simulink model "viatoc_run_sim"  (R2017b)
settings: Solver=FixedStepAuto  StartTime=0.0  StopTime=60  FixedStep=Ts  RelTol=1e-3
values from neighbouring files (symbols this model uses):
  Ts = 0.2    [U.mat]    (also in X.mat; hanging_chain_benchmark.m; num_iters.mat)
  u_0 = [-2 2 2]    [U.mat]    (also in X.mat; hanging_chain_benchmark.m = [-1; 1; 1]; num_iters.mat)
  x_0 = [1.875 0 0 3.75 0 0 5.625 0 0 7.5 0 0 ... (21 elements, 21x1)]    [U.mat]    (also in X.mat; num_iters.mat)
settings Model: Creator=robin  LastModifiedBy=robin

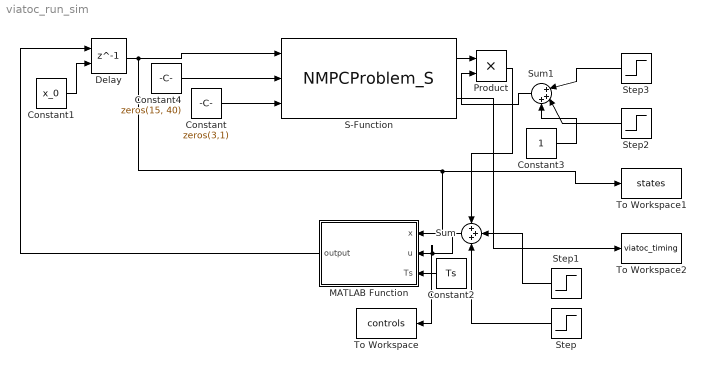
== system viatoc_run_sim ==
  Constant : Constant  Value=zeros(3,1)
  Constant1 : Constant  Value=x_0
  Constant2 : Constant  Value=Ts
  Constant3 : Constant
  Constant4 : Constant  Value=zeros(15, 40)  VectorParams1D=off
  Delay : Delay  DelayLength=1  InitialConditionSource=Input port
      settings: InputPortMap=u0,p4
  MATLAB Function : MATLAB Function  TreatAsAtomicUnit=on
  Product : Product
  S-Function : S-Function  FunctionName=NMPCProblem_S  SFunctionDeploymentMode=off  EnableBusSupport=off
  Step : Step  Time=29.8  Before=[0; 0; 0]  After=u_0  SampleTime=0
  Step1 : Step  Time=30.8  Before=[0; 0; 0]  After=-u_0  SampleTime=0
  Step2 : Step  Time=30.8  SampleTime=0
  Step3 : Step  Time=29.8  After=-1  SampleTime=0
  Sum : Sum  Inputs=+++
  Sum1 : Sum  Inputs=|+++
  To Workspace : ToWorkspace  VariableName=controls  SaveFormat=Timeseries  SampleTime=-1
  To Workspace1 : ToWorkspace  VariableName=states  SaveFormat=Timeseries  SampleTime=-1
  To Workspace2 : ToWorkspace  VariableName=viatoc_timing  SaveFormat=Timeseries  SampleTime=-1
  wires:
  Constant/1 -> S-Function/3
  Constant2/1 -> MATLAB Function/3(Ts)
  Constant4/1 -> S-Function/2
  Delay/1 -> To Workspace1/1, MATLAB Function/1(x), S-Function/1
  MATLAB Function/1(output) -> Delay/1
  Constant1/1 -> Delay/2
  S-Function/2 -> To Workspace2/1
  Sum/1 -> To Workspace/1, MATLAB Function/2(u)
  Step1/1 -> Sum/2
  Step/1 -> Sum/3
  Step2/1 -> Sum1/2
  Step3/1 -> Sum1/1
  S-Function/1 -> Product/1
  Sum1/1 -> Product/2
  Product/1 -> Sum/1
  Constant3/1 -> Sum1/3

== matlab function viatoc_run_sim/MATLAB Function ==
  data: x input; u input; output output; Ts input
function output = fcn(x, u, Ts)

[t_out, sim_out] = ode45(@(t, y) hanging_chain_ode(y, u, 3), [0 Ts], x);

output = zeros(21, 1);
for i=1:21
    output(i) = sim_out(end, i);
end
